simulink model "delays1"  (Simulink 9.2)
settings: Solver=ode45  StartTime=0.0  StopTime=10.0  RelTol=1e-3  EnableMultiTasking=on
settings Model: Creator=Jin  LastModifiedBy=jinwooro
settings DataIOCC: SignalLoggingSaveFormat=Dataset
settings DebuggingCC: SolverPrmCheckMsg=warning  FcnCallInpInsideContextMsg=error  StateNameClashWarn=none
settings GRTTargetCC: CombineOutputUpdateFcns=on  GRTInterface=off

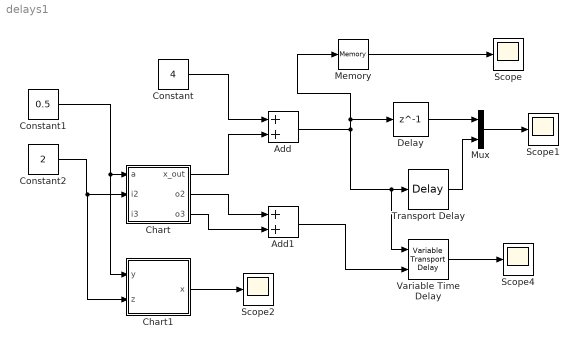
== system delays1 ==
  Add : Sum
  Add1 : Sum
  Chart : Stateflow chart  TreatAsAtomicUnit=on
  Chart1 : Stateflow chart  TreatAsAtomicUnit=on
  Constant : Constant  Value=4  OutDataTypeStr=double
  Constant1 : Constant  Value=0.5  OutMin=0  OutMax=3
  Constant2 : Constant  Value=2  OutMin=0  OutMax=3
  Delay : Delay  DelayLength=1  InitialCondition=0
  Memory : Memory
  Mux : Mux  Inputs=2
  Scope{,1..2,4} (4 alike) : Scope
  Transport Delay : TransportDelay
  Variable Time Delay : VariableTransportDelay  MaximumDelay=10
  wires:
  Constant/1 -> Add/1
  Add/1 -> Variable Time Delay/1, Transport Delay/1, Delay/1, Memory/1
  Chart/1(x_out) -> Add/2
  Constant1/1 -> Chart1/1(y), Chart/1(a)
  Constant2/1 -> Chart1/2(z), Chart/2(i2)
  Chart/2(o2) -> Add1/1
  Chart/3(o3) -> Add1/2
  Chart1/1(x) -> Scope2/1
  Memory/1 -> Scope/1
  Delay/1 -> Mux/1
  Mux/1 -> Scope1/1
  Transport Delay/1 -> Mux/2
  Add1/1 -> Variable Time Delay/2
  Variable Time Delay/1 -> Scope4/1

== stateflow chart Chart ==
  settings: updateMethod=CONTINUOUS
  state Init
    du:
    x_dot = a;
    x_out = x;
  state Finish
    du:
    x_dot = 0;
    x_out = x;
  (default) -> Init : {x = 1;}
  Init -> Finish : [x >= 7]
  data: x local double; x_out output double =3; a input double; y local double; o2 output double; i2 input double; o3 output double; i3 input double
  data x settings: updateMethod=SF_CONTINUOUS_TIME_DATA

== stateflow chart Chart1 ==
  state Hi
    du:
    x = y + z;
  (default) -> Hi
  data: x output double; y input double; z input double
